simulink model "example_rotor_estimation"  (R2016a)
settings: Solver=VariableStepAuto  StartTime=0.0  StopTime=20  RelTol=1e-3
settings Model: Creator=mgreiff  LastModifiedBy=mgreiff

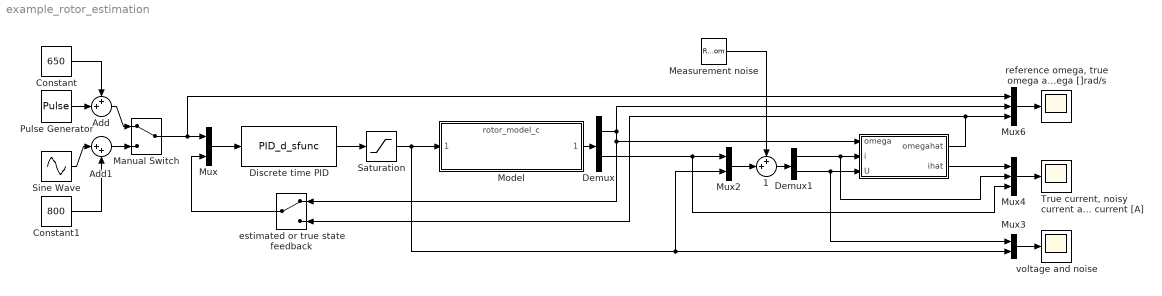
== system example_rotor_estimation ==
  "      " : Subsystem
  "    1" : Sum  Inputs=++|
  " reference omega, true omega and estimated omega []rad/s" : Scope
  Add : Sum  Inputs=++|
  Add1 : Sum  Inputs=|++
  Constant : Constant  Value=650
  Constant1 : Constant  Value=800
  Demux : Demux  Outputs=2
  Demux1 : Demux  Outputs=2
  Discrete time PID : S-Function  FunctionName=PID_d_sfunc  Parameters=PIDparam  SFunctionDeploymentMode=off  EnableBusSupport=off
  Manual Switch : ManualSwitch
  Measurement noise : RandomNumber  Mean=[0,0]  Variance=[0.001, 0.001]  Seed=1
  Model : ModelReference  ModelNameDialog=rotor_model_c.slx  SimulationMode=Normal  ModelReferenceVersion=1.28
  Mux : Mux  Inputs=2
  Mux2 : Mux  Inputs=2
  Mux3 : Mux  Inputs=2
  Mux4 : Mux  Inputs=3
  Mux6 : Mux  Inputs=3
  Pulse Generator : DiscretePulseGenerator  PulseType=Time based  Amplitude=600  Period=4  PulseWidth=50
  Saturation : Saturate  UpperLimit=4.3  LowerLimit=0
  Sine Wave : Sin  Amplitude=300  Frequency=0.5  SampleTime=0
  "True current, noisy current and estimated current [A]  " : Scope
  estimated or true state feedback : ManualSwitch
  voltage and noise : Scope
  wires:
  Model/1 -> Demux/1
  Mux/1 -> Discrete time PID/1
  Manual Switch/1 -> Mux6/1, Mux/1
  Constant/1 -> Add/1
  Discrete time PID/1 -> Saturation/1
  Demux/2 -> Mux4/3, Mux2/1
  Add/1 -> Manual Switch/1
  Pulse Generator/1 -> Add/2
  Sine Wave/1 -> Add1/1
  Add1/1 -> Manual Switch/2
  Constant1/1 -> Add1/2
  Mux3/1 -> voltage and noise/1
  Mux4/1 -> "True current, noisy current and estimated current [A]  "/1
  Mux6/1 -> " reference omega, true omega and estimated omega []rad/s"/1
  Saturation/1 -> Mux2/2, Mux3/2, Model/1
  "      "/1(omegahat) -> estimated or true state feedback/2, Mux6/3
  Demux1/2 -> Mux3/1, "      "/3(U)
  Demux1/1 -> Mux4/2, "      "/2(i)
  estimated or true state feedback/1 -> Mux/2
  Mux2/1 -> "    1"/2
  "    1"/1 -> Demux1/1
  Measurement noise/1 -> "    1"/1
  "      "/2(ihat) -> Mux4/1
  Demux/1 -> "      "/1(omega), estimated or true state feedback/1, Mux6/2

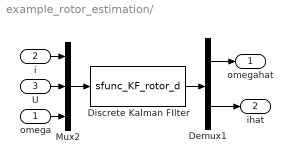
== system example_rotor_estimation/       ==
  omega : Inport
  i : Inport  Port=2
  U : Inport  Port=3
  Demux1 : Demux  Outputs=2
  Discrete Kalman FIlter : S-Function  FunctionName=sfunc_KF_rotor_d  Parameters=FILTERparam  SFunctionDeploymentMode=off  EnableBusSupport=off
  Mux2 : Mux  Inputs=3
  omegahat : Outport
  ihat : Outport  Port=2
  wires:
  i/1 -> Mux2/1
  Demux1/2 -> ihat/1
  Demux1/1 -> omegahat/1
  Discrete Kalman FIlter/1 -> Demux1/1
  Mux2/1 -> Discrete Kalman FIlter/1
  omega/1 -> Mux2/3
  U/1 -> Mux2/2
